simulink model "test_model"  (R2022b)
settings: Solver=VariableStepAuto  StartTime=0.0  StopTime=10.0  RelTol=1e-3
libraries: gmp_sil_core_pack x1
settings Model: Creator=javnson  LastModifiedBy=javnson

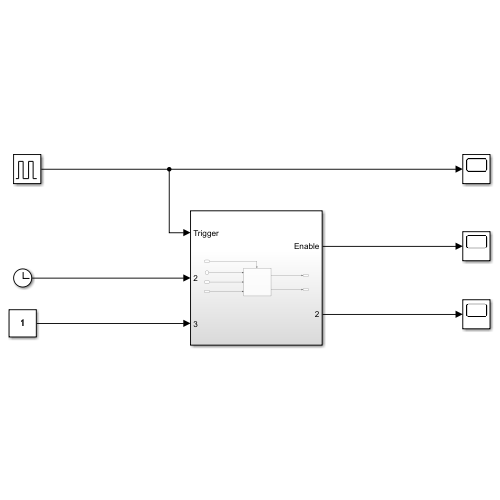
[thumbnail: Simulink's stored preview of the top-level diagram]
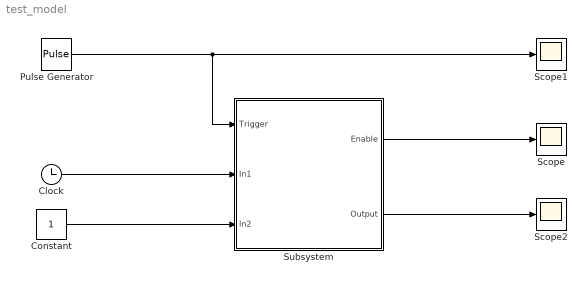
== system test_model ==
  Clock : Clock
  Constant : Constant
  Pulse Generator : DiscretePulseGenerator  PulseType=Time based  Period=0.1  PulseWidth=5
  Scope : Scope
  Scope1 : Scope
  Scope2 : Scope
  Subsystem : Subsystem
  wires:
  Clock/1 -> Subsystem/2(In1)
  Constant/1 -> Subsystem/3(In2)
  Subsystem/1(Enable) -> Scope/1
  Pulse Generator/1 -> Scope1/1, Subsystem/1(Trigger)
  Subsystem/2(Output) -> Scope2/1

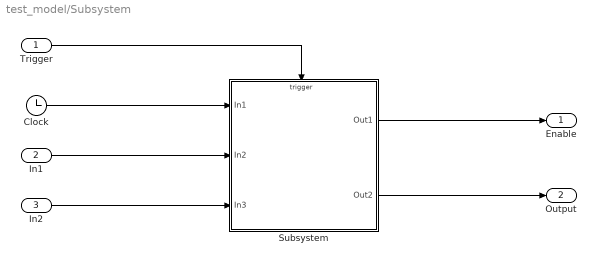
== system test_model/Subsystem ==
  Trigger : Inport
  In1 : Inport  Port=2
  In2 : Inport  Port=3
  Clock : Clock
  Subsystem : Subsystem
  Enable : Outport
  Output : Outport  Port=2
  wires:
  Clock/1 -> Subsystem/1(In1)
  In1/1 -> Subsystem/2(In2)
  In2/1 -> Subsystem/3(In3)
  Subsystem/1(Out1) -> Enable/1
  Subsystem/2(Out2) -> Output/1
  Trigger/1 -> Subsystem/Trigger

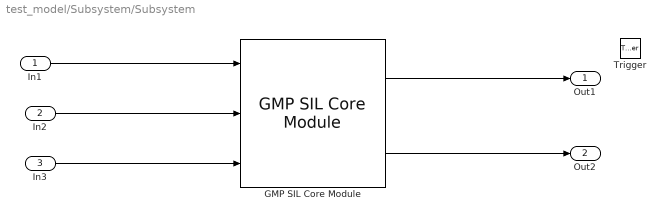
== system test_model/Subsystem/Subsystem ==
  In1 : Inport
  In2 : Inport  Port=2
  In3 : Inport  Port=3
  Trigger : TriggerPort  VariantControl=(inherit)  PortDimensions=1
  GMP SIL Core Module : gmp_sil_core_pack/GMP SIL Core Module  MaskPackedDataTypes={'double','double','double'}  MaskPackedDataSizes={[1],[1],[1]}  MaskUnpackedDataTypes={'double','double'}  MaskUnpackedDataSizes={[1],[1]}  MaskAlignment=1  MaskHostAddr='127.0.0.1'  MaskMsgTxPort=12300  MaskMsgRxPort=12301  MaskCmdTxPort=12302  MaskCmdRxPort=12303
      settings: SourceProductName=GMP Utilities Library
  Out1 : Outport
  Out2 : Outport  Port=2
  wires:
  GMP SIL Core Module/1 -> Out1/1
  In1/1 -> GMP SIL Core Module/1
  In2/1 -> GMP SIL Core Module/2
  In3/1 -> GMP SIL Core Module/3
  GMP SIL Core Module/2 -> Out2/1
